simulink model "sogi_dual_output_filter_fe_discrete"  (R2026a)
settings: Solver=FixedStepDiscrete  StopTime=1
settings Model: DataDictionary=sogi_state_space_parameters.sldd  EnableAccessToBaseWorkspace=off  Creator=ASUS  LastModifiedBy=ASUS

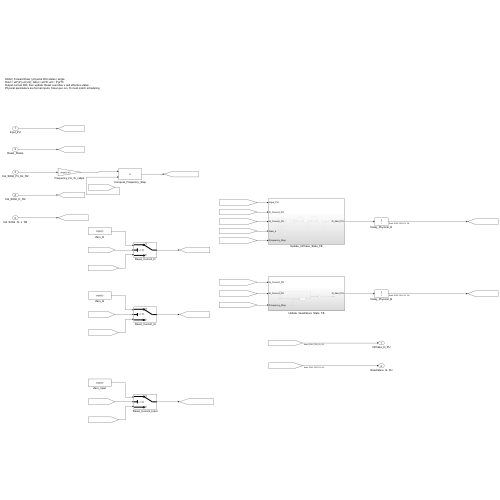
[thumbnail: Simulink's stored preview of the top-level diagram]
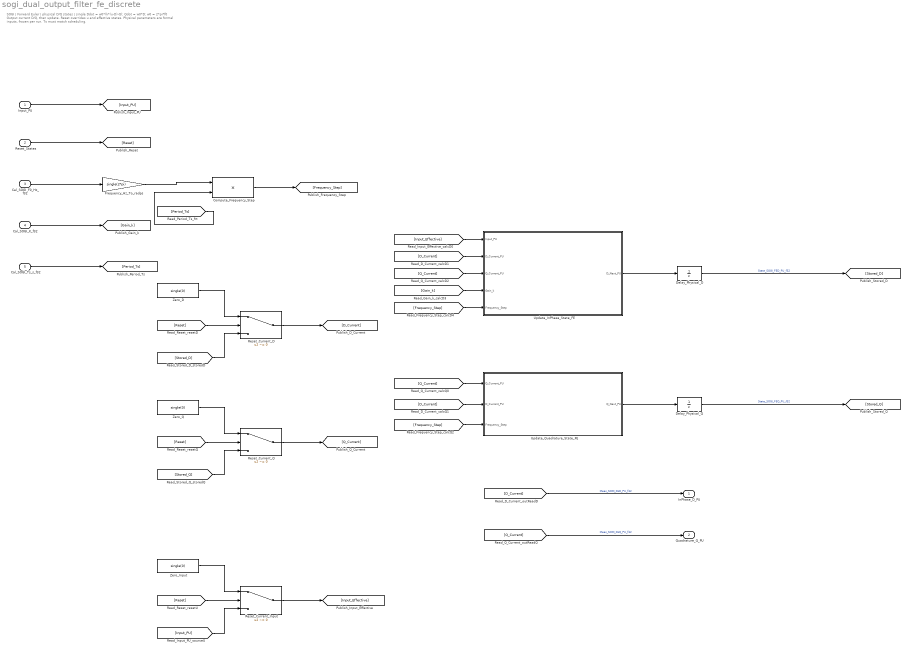
== system sogi_dual_output_filter_fe_discrete ==
  note: SOGI | Forward Euler | physical D/Q states | single
      | Ddot = w0*(k*(u-D)-Q); Qdot = w0*D; w0 = 2*pi*f0
      | Output current D/Q, then update. Reset overrides u and effective states.
      | Physical parameters are formal inputs, frozen per run. Ts must match scheduling.
  Input_PU : Inport  OutDataTypeStr=single  PortDimensions=1  Interpolate=off
  Reset_States : Inport  Port=2  OutDataTypeStr=uint8  PortDimensions=1  Interpolate=off
  Cal_SOGI_F0_Hz_f32 : Inport  Port=3  OutDataTypeStr=single  PortDimensions=1  Interpolate=off
  Cal_SOGI_K_f32 : Inport  Port=4  OutDataTypeStr=single  PortDimensions=1  Interpolate=off
  Cal_SOGI_Ts_s_f32 : Inport  Port=5  OutDataTypeStr=single  PortDimensions=1  Interpolate=off
  Compute_Frequency_Step : Product  Inputs=**  OutDataTypeStr=single
  Delay_Physical_D : UnitDelay  InitialCondition=single(0)  SampleTime=-1
  Delay_Physical_Q : UnitDelay  InitialCondition=single(0)  SampleTime=-1
  Frequency_Hz_To_radps : Gain  Gain=single(2*pi)  ParamDataTypeStr=single  OutDataTypeStr=single
  Reset_Current_D : Switch  Criteria=u2 ~= 0  OutDataTypeStr=single  SaturateOnIntegerOverflow=off  InputSameDT=off
  Reset_Current_Input : Switch  Criteria=u2 ~= 0  OutDataTypeStr=single  SaturateOnIntegerOverflow=off  InputSameDT=off
  Reset_Current_Q : Switch  Criteria=u2 ~= 0  OutDataTypeStr=single  SaturateOnIntegerOverflow=off  InputSameDT=off
  Update_InPhase_State_FE : Subsystem
  Update_Quadrature_State_FE : Subsystem
  Zero_D : Constant  Value=single(0)  OutDataTypeStr=single  SampleTime=-1
  Zero_Input : Constant  Value=single(0)  OutDataTypeStr=single  SampleTime=-1
  Zero_Q : Constant  Value=single(0)  OutDataTypeStr=single  SampleTime=-1
  InPhase_D_PU : Outport  OutDataTypeStr=single  PortDimensions=1
  Quadrature_Q_PU : Outport  Port=2  OutDataTypeStr=single  PortDimensions=1
  wires:
  [Q_Current] -> Quadrature_Q_PU/1  "Meas_SOGI_FEQ_PU_f32"
  Delay_Physical_Q/1 -> [Stored_Q]  "State_SOGI_FEQ_PU_f32"
  Update_Quadrature_State_FE/1(Q_Next_PU) -> Delay_Physical_Q/1
  [Frequency_Step] -> Update_Quadrature_State_FE/3(Frequency_Step)
  [D_Current] -> Update_Quadrature_State_FE/2(D_Current_PU)
  [Q_Current] -> Update_Quadrature_State_FE/1(Q_Current_PU)
  [D_Current] -> InPhase_D_PU/1  "Meas_SOGI_FED_PU_f32"
  Delay_Physical_D/1 -> [Stored_D]  "State_SOGI_FED_PU_f32"
  Update_InPhase_State_FE/1(D_Next_PU) -> Delay_Physical_D/1
  [Frequency_Step] -> Update_InPhase_State_FE/5(Frequency_Step)
  [Gain_k] -> Update_InPhase_State_FE/4(Gain_k)
  [Q_Current] -> Update_InPhase_State_FE/3(Q_Current_PU)
  [D_Current] -> Update_InPhase_State_FE/2(D_Current_PU)
  [Input_Effective] -> Update_InPhase_State_FE/1(Input_PU)
  Reset_Current_Input/1 -> [Input_Effective]
  [Input_PU] -> Reset_Current_Input/3
  [Reset] -> Reset_Current_Input/2
  Zero_Input/1 -> Reset_Current_Input/1
  Reset_Current_Q/1 -> [Q_Current]
  [Stored_Q] -> Reset_Current_Q/3
  [Reset] -> Reset_Current_Q/2
  Zero_Q/1 -> Reset_Current_Q/1
  Reset_Current_D/1 -> [D_Current]
  [Stored_D] -> Reset_Current_D/3
  [Reset] -> Reset_Current_D/2
  Zero_D/1 -> Reset_Current_D/1
  Compute_Frequency_Step/1 -> [Frequency_Step]
  [Period_Ts] -> Compute_Frequency_Step/2
  Frequency_Hz_To_radps/1 -> Compute_Frequency_Step/1
  Cal_SOGI_F0_Hz_f32/1 -> Frequency_Hz_To_radps/1
  Cal_SOGI_Ts_s_f32/1 -> [Period_Ts]
  Cal_SOGI_K_f32/1 -> [Gain_k]
  Reset_States/1 -> [Reset]
  Input_PU/1 -> [Input_PU]

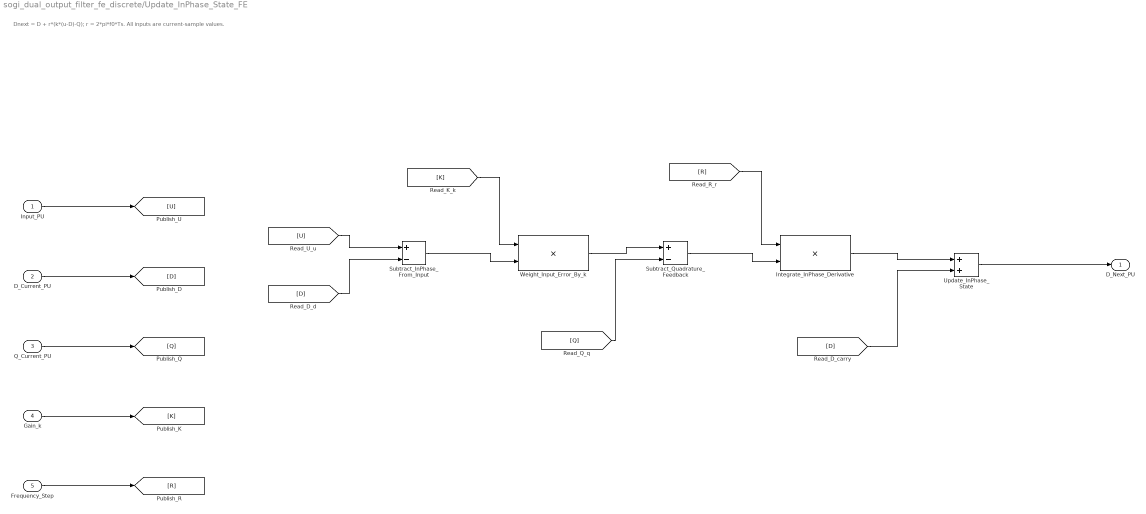
== system sogi_dual_output_filter_fe_discrete/Update_InPhase_State_FE ==
  note: Dnext = D + r*(k*(u-D)-Q); r = 2*pi*f0*Ts. All inputs are current-sample values.
  Input_PU : Inport  OutDataTypeStr=single  PortDimensions=1
  D_Current_PU : Inport  Port=2  OutDataTypeStr=single  PortDimensions=1
  Q_Current_PU : Inport  Port=3  OutDataTypeStr=single  PortDimensions=1
  Gain_k : Inport  Port=4  OutDataTypeStr=single  PortDimensions=1
  Frequency_Step : Inport  Port=5  OutDataTypeStr=single  PortDimensions=1
  Integrate_InPhase_Derivative : Product  Inputs=**  OutDataTypeStr=single
  Subtract_InPhase_From_Input : Sum  Inputs=+-  OutDataTypeStr=single
  Subtract_Quadrature_Feedback : Sum  Inputs=+-  OutDataTypeStr=single
  Update_InPhase_State : Sum  OutDataTypeStr=single
  Weight_Input_Error_By_k : Product  Inputs=**  OutDataTypeStr=single
  D_Next_PU : Outport  OutDataTypeStr=single  PortDimensions=1
  wires:
  Update_InPhase_State/1 -> D_Next_PU/1
  [D] -> Update_InPhase_State/2
  Integrate_InPhase_Derivative/1 -> Update_InPhase_State/1
  Subtract_Quadrature_Feedback/1 -> Integrate_InPhase_Derivative/2
  [R] -> Integrate_InPhase_Derivative/1
  [Q] -> Subtract_Quadrature_Feedback/2
  Weight_Input_Error_By_k/1 -> Subtract_Quadrature_Feedback/1
  Subtract_InPhase_From_Input/1 -> Weight_Input_Error_By_k/2
  [K] -> Weight_Input_Error_By_k/1
  [D] -> Subtract_InPhase_From_Input/2
  [U] -> Subtract_InPhase_From_Input/1
  Frequency_Step/1 -> [R]
  Gain_k/1 -> [K]
  Q_Current_PU/1 -> [Q]
  D_Current_PU/1 -> [D]
  Input_PU/1 -> [U]

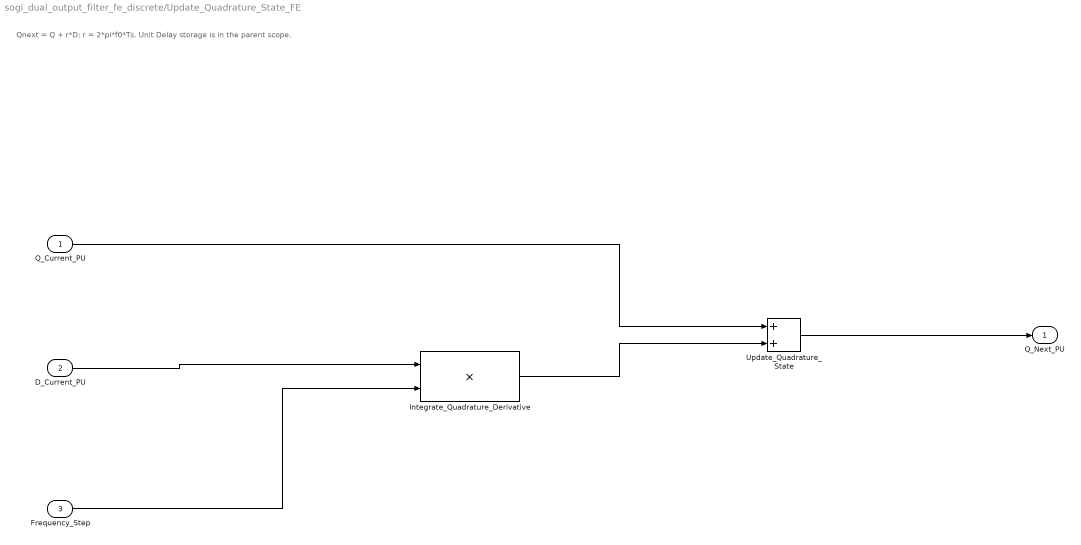
== system sogi_dual_output_filter_fe_discrete/Update_Quadrature_State_FE ==
  note: Qnext = Q + r*D; r = 2*pi*f0*Ts. Unit Delay storage is in the parent scope.
  Q_Current_PU : Inport  OutDataTypeStr=single  PortDimensions=1
  D_Current_PU : Inport  Port=2  OutDataTypeStr=single  PortDimensions=1
  Frequency_Step : Inport  Port=3  OutDataTypeStr=single  PortDimensions=1
  Integrate_Quadrature_Derivative : Product  Inputs=**  OutDataTypeStr=single
  Update_Quadrature_State : Sum  OutDataTypeStr=single
  Q_Next_PU : Outport  OutDataTypeStr=single  PortDimensions=1
  wires:
  Update_Quadrature_State/1 -> Q_Next_PU/1
  Integrate_Quadrature_Derivative/1 -> Update_Quadrature_State/2
  Q_Current_PU/1 -> Update_Quadrature_State/1
  Frequency_Step/1 -> Integrate_Quadrature_Derivative/2
  D_Current_PU/1 -> Integrate_Quadrature_Derivative/1
